simulink model "hamiltonian_data_collector"  (R2012b)
settings: Solver=ode3  StartTime=0.0  StopTime=10  FixedStep=0.01  RelTol=1e-3
settings Model: ExtModeTrigDuration=5000  Creator=crbonney  LastModifiedBy=crbonney
settings SolverCC: PositivePriorityOrder=on
settings RTWCC: SystemTargetFile=quarc_win64.tlc  TemplateMakefile=quarc_default_tmf  Description=QUARC Win64 Target  ProcessScript=quarc_win64_make_rtw_hook
settings STFCustomTargetCC: TargetPreCompLibLocation=C:\PROGRA~3\QUARC\lib\2012b\win64\release  CodeReplacementLibrary=ANSI_C  GeneratePreprocessorConditionals=Disable all  CombineOutputUpdateFcns=on  GRTInterface=off  SystemTargetFile=quarc_win64.tlc
settings GRTTargetCC: TargetPreCompLibLocation=C:\PROGRA~3\QUARC\lib\2012b\win64\release  ParMdlRefBuildCompliant=off  CompOptLevelCompliant=off  ConcurrentExecutionCompliant=off  MatFileLogging=off  ExtMode=on  ExtModeMexFile=quarc_comm

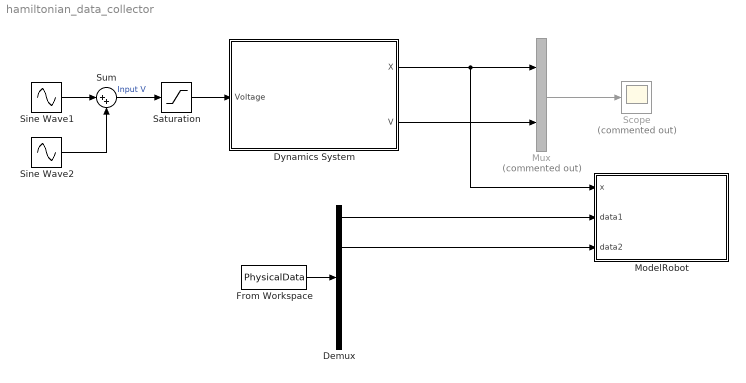
== system hamiltonian_data_collector ==
  Demux : Demux  Outputs=5
  Dynamics System : Subsystem
  From Workspace : FromWorkspace  VariableName=PhysicalData  SampleTime=0
  ModelRobot : MATLAB Function  TreatAsAtomicUnit=on
  Mux : Mux  Commented=on  Inputs=2
  Saturation : Saturate  UpperLimit=10  LowerLimit=-10
  Scope : Scope  Commented=on
      settings: SaveName=SimulationData  MaxDataPoints=10000
  Sine Wave1 : Sin  Amplitude=4  Frequency=5
  Sine Wave2 : Sin  Amplitude=4  Frequency=15
  Sum : Sum  Inputs=|++
  wires:
  Dynamics System/1(X) -> ModelRobot/1(x), Mux/1
  Dynamics System/2(V) -> Mux/2
  Mux/1 -> Scope/1
  Saturation/1 -> Dynamics System/1(Voltage)
  Sum/1 -> Saturation/1  "Input V"
  Sine Wave1/1 -> Sum/1
  Sine Wave2/1 -> Sum/2
  From Workspace/1 -> Demux/1
  Demux/1 -> ModelRobot/2(data1)
  Demux/2 -> ModelRobot/3(data2)

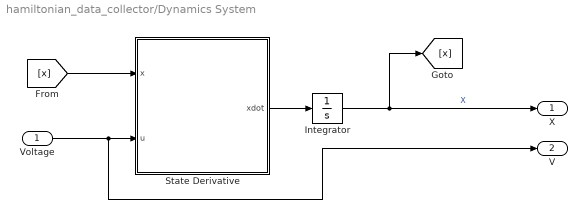
== system hamiltonian_data_collector/Dynamics System ==
  Voltage : Inport
  Integrator : Integrator  InitialCondition=[0;pi;0;0]
  State Derivative : MATLAB Function  TreatAsAtomicUnit=on
  X : Outport
  V : Outport  Port=2
  wires:
  State Derivative/1(xdot) -> Integrator/1
  Voltage/1 -> V/1, State Derivative/2(u)
  [x] -> State Derivative/1(x)
  Integrator/1 -> X/1, [x]  "X"

== matlab function hamiltonian_data_collector/ModelRobot ==
  data: x input; data1 input; data2 input
function ModelRobot (x,data1,data2)

theta1 = x(1);
theta2 = x(2);

    frame0_links = ...
        [0  0;...  %X
         0  0;...  %Y
         0 -15];   %Z

    frame1_links = ...
        [0  0  0  0 0;... %X
         0  0  6  6 8;... %Y
         0 -1 -1  0 0];   %Z

    frame2_links = ...
        [0   0;... %X
         0  12;... %Y
         0   0];   %Z

    rho = sqrt(8^2+12^2);
    phi_max = atan(12/8);

    f1 = TransformPoints(TRANS0_1(theta1),frame1_links);
    f2 = TransformPoints(TRANS0_1(theta1),TransformPoints(TRANS1_2(theta2),frame2_links));
    d1 = TransformPoints(TRANS0_1(data1),frame1_links);
    d2 = TransformPoints(TRANS0_1(data1),TransformPoints(TRANS1_2(data2),frame2_links));    

    plot3(frame0_links(1,:),frame0_links(2,:), frame0_links(3,:),'bs-','LineWidth',3);
    axis([-15 15 -15 15 -15 15]);
    grid on
    hold on
    xlabel('x');
    ylabel('y');
    zlabel('z');
    plot3(f1(1,:),f1(2,:), f1(3,:),'rs-','LineWidth',3);
    plot3(f2(1,:),f2(2,:), f2(3,:),'go-', 'MarkerFaceColor', 'c', 'MarkerSize',5,'LineWidth',3);
    plot3(f2(1,end),f2(2,end), f2(3,end),'go-', 'MarkerFaceColor', 'c', 'MarkerSize',5,'LineWidth',3);

    plot3(d1(1,:),d1(2,:), d1(3,:),'ks-','LineWidth',3);
    plot3(d2(1,:),d2(2,:), d2(3,:),'ko-', 'MarkerFaceColor', 'k', 'MarkerSize',5,'LineWidth',3);
    plot3(d2(1,end),d2(2,end), d2(3,end),'ko-', 'MarkerFaceColor', 'k', 'MarkerSize',5,'LineWidth',3);

    axis([-15 15 -15 15 -15 15]);
    WorkEnvelope2(rho, phi_max);
    hold off
end

== matlab function hamiltonian_data_collector/Dynamics System/State Derivative ==
  data: x input; u input; xdot output
function xdot = fcn(x, u)

%% constants
% J1 = 0.0012;
% m2 = 0.127;
% L12 = 0.2;
% L2 = 0.3;
% Lc2 = L2/2;
% beta1 = 0.015;
% beta2 = 0.002;
% Ra = 2.6;
% kt = 0.00768;
% kr = 70;
g = 9.81;
% 
%% parameters
% theta1 = (J1+m2*L12^2)*Ra/(kr*kt);
% theta2 = 1/3*m2*L2^2*Ra/(kr*kt);
% theta3 = 1/2*m2*L12*L2*Ra/(kr*kt);
% theta4 = m2*Lc2*Ra/(kr*kt);
% theta5 = beta1*Ra/(kr*kt)+kr*kt;
% theta6 = beta2*Ra/(kr*kt);

% CALCULATED THETAS
% theta1 = 0.030372023809524;
% theta2 = 0.018426339285714;
% theta3 = 0.018426339285714;
% theta4 = 0.092131696428571;
% theta5 = 0.610144642857143;
% theta6 = 0.009672619047619;

% HAMILTONIAN THETAS
theta1 = 0.089626860251478;
theta2 = 0.027476488534314;
theta3 = 0.029103291131862;
theta4 = 0.114763241730839;
theta5 = 0.560169997835625;
theta6 = 0.011135861988403;

%% unpack vector
q1 = x(1);
q2 = x(2);
q1dot = x(3);
q2dot = x(4);
v = [-u; 0];

%% make matrices
m =    [...
        (theta1+theta2*sin(q2)^2)   (theta3*cos(q2)) ;...
            (theta3*cos(q2))            (theta2)     ;...
];


c =    [...
        (2*theta2*sin(q2)*cos(q2)*q2dot)     (-theta3*sin(q2)*q2dot) ;...
         (-theta2*sin(q2)*cos(q2)*q1dot)               (0)           ;...
];


f =    [...
         theta5*q1dot;...
         theta6*q2dot;...
];

g =    [...
                0         ;...
        -theta4*g*sin(q2) ;...
];

%% get accleration
acceleration = -m\(c*[q1dot;q2dot]+f+g-v);

%% get state derivative
xdot = [q1dot;q2dot;acceleration];
% xdot = [q1dot; q2dot; q1ddot; q2ddot];
